simulink model "EngReq_TrqLimCalc"  (R2016b)
settings: configuration reference "CodeGenConfigSet" (kept outside this file)
settings Model: Creator=Administrator  LastModifiedBy=Wei Liang
settings ConfigSetRef: SourceLocation=Base Workspace

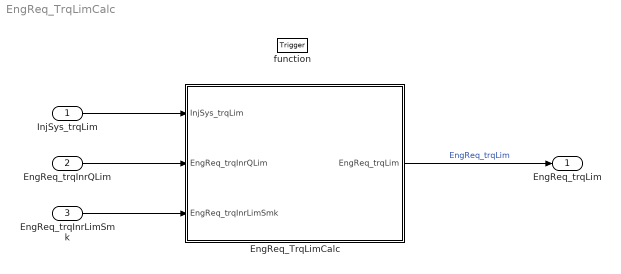
== system EngReq_TrqLimCalc ==
  InjSys_trqLim : Inport  Tag=Nm  Description=Torque limitation of injection system  OutMin=-3276.8  OutMax=3276.7  OutDataTypeStr=Trq_Nm
  EngReq_trqInrQLim : Inport  Tag=Nm  Description=Limiting torque due to limitation quantities (except smoke limitation)  Port=2  OutMin=-3276.8  OutMax=3276.7  OutDataTypeStr=Trq_Nm
  EngReq_trqInrLimSmk : Inport  Tag=Nm  Description=Limiting torque smoke limit  Port=3  OutMin=-3276.8  OutMax=3276.7  OutDataTypeStr=Trq_Nm
  function : TriggerPort  TriggerType=function-call  VariantControl=Variant
  EngReq_TrqLimCalc : Subsystem
  EngReq_trqLim : Outport  Tag=Nm  Description=Resulting limiting torque from engine specifications  OutMin=-3276.8  OutMax=3276.7  OutDataTypeStr=Trq_Nm
  wires:
  InjSys_trqLim/1 -> EngReq_TrqLimCalc/1(InjSys_trqLim)
  EngReq_trqInrQLim/1 -> EngReq_TrqLimCalc/2(EngReq_trqInrQLim)
  EngReq_trqInrLimSmk/1 -> EngReq_TrqLimCalc/3(EngReq_trqInrLimSmk)
  EngReq_TrqLimCalc/1(EngReq_trqLim) -> EngReq_trqLim/1  "EngReq_trqLim"

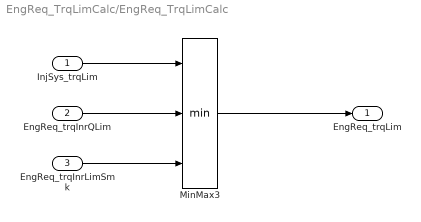
== system EngReq_TrqLimCalc/EngReq_TrqLimCalc ==
  InjSys_trqLim : Inport  Tag=Nm  Description=Torque limitation of injection system  OutMin=-3276.8  OutMax=3276.7  OutDataTypeStr=Trq_Nm
  EngReq_trqInrQLim : Inport  Tag=Nm  Description=Limiting torque due to limitation quantities (except smoke limitation)  Port=2  OutMin=-3276.8  OutMax=3276.7  OutDataTypeStr=Trq_Nm
  EngReq_trqInrLimSmk : Inport  Tag=Nm  Description=Limiting torque smoke limit  Port=3  OutMin=-3276.8  OutMax=3276.7  OutDataTypeStr=Trq_Nm
  MinMax3 : MinMax  Inputs=3  InputSameDT=on
  EngReq_trqLim : Outport  Tag=Nm  Description=Torque limitation due to engine requests  OutMin=-3276.8  OutMax=3276.7  OutDataTypeStr=Trq_Nm
  wires:
  MinMax3/1 -> EngReq_trqLim/1
  InjSys_trqLim/1 -> MinMax3/1
  EngReq_trqInrQLim/1 -> MinMax3/2
  EngReq_trqInrLimSmk/1 -> MinMax3/3
